simulink model "LQR_CO_NHIEU"  (R2017b)
settings: Solver=FixedStepAuto  StartTime=0.0  StopTime=30  FixedStep=0.01  RelTol=1e-3
values from neighbouring files (symbols this model uses):
  K = lqr(A,B,Q,R__)    [CacFunctionTrongSimulink_LQR.m]    (also in QQQQ.m = lqr(A,B,Q,R); TINHGIATRIK.m = lqr(A,B,Q,R); TINHTHONGSOLQG.m = lqr(A,B,Q,R))
libraries: simulink x2
settings Model: Creator=DELL  LastModifiedBy=DELL

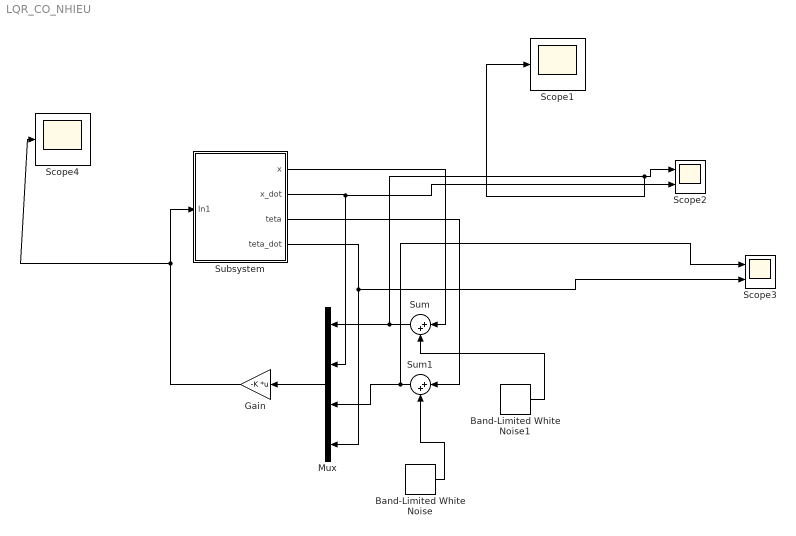
== system LQR_CO_NHIEU ==
  Band-Limited White Noise : simulink/Sources/Band-Limited White Noise  Cov=[0.0000001]  Ts=0.01  seed=[23341]
  Band-Limited White Noise1 : simulink/Sources/Band-Limited White Noise  Cov=[0.000001]  Ts=0.01  seed=[23341]
  Gain : Gain  Gain=-K  Multiplication=Matrix(K*u)
  Mux : Mux
  Scope1 : Scope
  Scope2 : Scope  NumInputPorts=2
  Scope3 : Scope  NumInputPorts=2
  Scope4 : Scope
  Subsystem : Subsystem
  Sum : Sum  Inputs=|++
  Sum1 : Sum  Inputs=|++
  wires:
  Gain/1 -> Scope4/1, Subsystem/1(In1)
  Mux/1 -> Gain/1
  Sum/1 -> Scope1/1, Scope2/1, Mux/1
  Subsystem/1(x) -> Sum/1
  Band-Limited White Noise1/1 -> Sum/2
  Subsystem/3(teta) -> Sum1/1
  Band-Limited White Noise/1 -> Sum1/2
  Sum1/1 -> Scope3/1, Mux/3
  Subsystem/2(x_dot) -> Scope2/2, Mux/2
  Subsystem/4(teta_dot) -> Scope3/2, Mux/4

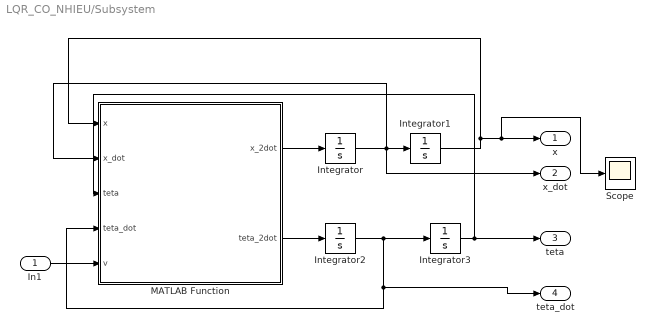
== system LQR_CO_NHIEU/Subsystem ==
  In1 : Inport
  Integrator : Integrator
  Integrator1 : Integrator  InitialCondition=0.05
  Integrator2 : Integrator
  Integrator3 : Integrator  InitialCondition=0.05
  MATLAB Function : MATLAB Function  TreatAsAtomicUnit=on
  Scope : Scope
  x : Outport
  x_dot : Outport  Port=2
  teta : Outport  Port=3
  teta_dot : Outport  Port=4
  wires:
  In1/1 -> MATLAB Function/5(v)
  Integrator/1 -> x_dot/1, MATLAB Function/2(x_dot), Integrator1/1
  MATLAB Function/1(x_2dot) -> Integrator/1
  Integrator3/1 -> teta/1, MATLAB Function/3(teta)
  MATLAB Function/2(teta_2dot) -> Integrator2/1
  Integrator1/1 -> x/1, Scope/1, MATLAB Function/1(x)
  Integrator2/1 -> teta_dot/1, MATLAB Function/4(teta_dot), Integrator3/1

== matlab function LQR_CO_NHIEU/Subsystem/MATLAB Function ==
  data: x input; x_2dot output; x_dot input; teta input; teta_dot input; v input; teta_2dot output
function [x_2dot,teta_2dot] = fcn(x,x_dot,teta,teta_dot,v)

g=9.81; %Gravity(m/s^2)
r=0.051; %Radius of wheel(m)
Mw=0.03; %Mass of wheel(kg)
Mp=1.13; %Mass of body(kg)
Iw=0.000039; %Inertia of the wheel(kg*m^2)
Ip=0.0041; %Inertia of the body(kg*m^2)
L=0.07; %Length to the body's center of mass(m)

%Motor's variables
Km=0.006123; %Motor torque constant(Nm/A)
Ke=0.006087; %Back EMF constant(Vs/rad)
R=3; %Nominal terminal resistance(Ohm)
a1=Mp*L/(Ip+Mp*L^2);
a2=Km*Ke/(R*r*(Ip+Mp*L^2));
a3=Km/(R*(Ip+Mp*L^2));
a4=Mp*g*L/(Ip+Mp*L^2);
b1=2*Km/(R*r*(2*Mw+2*(Iw/r^2)+Mp));
b2=2*Km*Ke/(R*r^2*(2*Mw+2*(Iw/r^2)+Mp));
b3=Mp*L/(2*Mw+2*(Iw/r^2)+Mp);
K=1.0e+03 *[-0.0316   -0.0361    1.6415    0.1272];
teta_2dot = -(a4*teta - 2*a3*v + 2*a2*x + a1*b1*v - a1*b2*x_dot)/(a1*b3 - 1);
x_2dot=-(b1*v - b2*x_dot + a4*b3*teta - 2*a3*b3*v + 2*a2*b3*x)/(a1*b3 - 1);
